simulink model "kaskadydolinearyzacjimud6"  (R2019b)
settings: Solver=VariableStepAuto  StartTime=0.0  StopTime=150  RelTol=1e-3
values from neighbouring files (symbols this model uses):
  A1 = 1    [linearyzacjamud6.m]
  a1 = Aw1*sqrt(2*g)    [linearyzacjamud6.m]
  A2 = 1    [linearyzacjamud6.m]
  a2 = Aw2*sqrt(2*g)    [linearyzacjamud6.m]
  fwe = 0.7*fwemax    [linearyzacjamud6.m]
  fwe0 = 0.1*fwemax    [linearyzacjamud6.m]
  h1pocz = fwe0/a1    [linearyzacjamud6.m]
  h2pocz = fwe0/a2    [linearyzacjamud6.m]
settings Model: Creator=tomek  LastModifiedBy=tomek

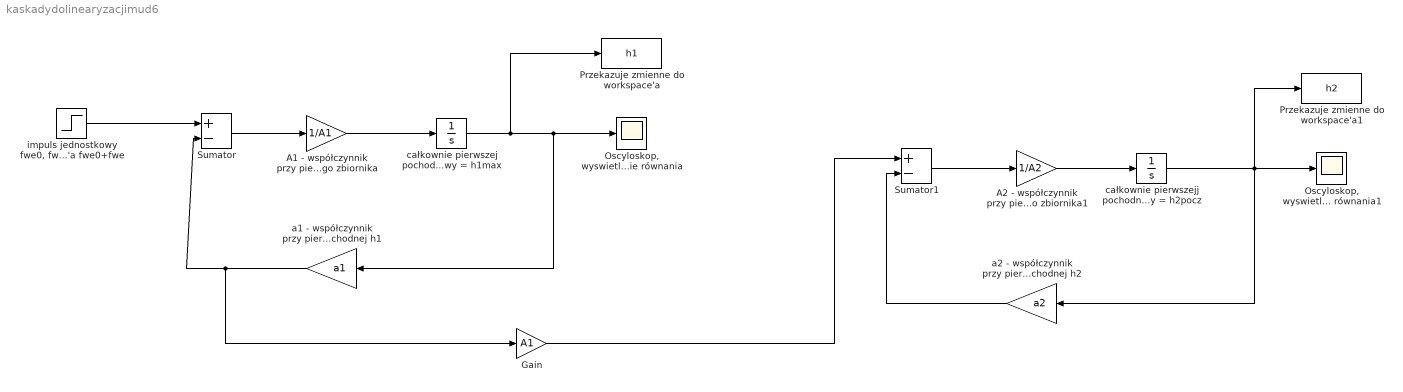
== system kaskadydolinearyzacjimud6 ==
  " całkownie pierwszej pochodnej h1, zawiera warunki początkowe warunek początkowy = h1max" : Integrator  InitialCondition=h1pocz
  " całkownie pierwszejj pochodnej h2 zawiera warunki początkowe warunek poczatkowy = h2pocz" : Integrator  InitialCondition=h2pocz
  A1 - współczynnik przy pierwszej pchodnej h1 Powierzchnia dna pierwszego zbiornika : Gain  Gain=1/A1
  A2 - współczynnik przy pierwszej pchodnej h2 Powierzchnia dna pierwszego zbiornika1 : Gain  Gain=1/A2
  Gain : Gain  Gain=A1
  "Oscyloskop, wyswietla roziwązanie równania" : Scope
  "Oscyloskop, wyswietla roziwązanie równania1" : Scope
  Przekazuje zmienne do workspace'a : ToWorkspace  VariableName=h1  SampleTime=-1
  Przekazuje zmienne do workspace'a1 : ToWorkspace  VariableName=h2  SampleTime=-1
  Sumator : Sum  Inputs=+-
  Sumator1 : Sum  Inputs=+-
  a1 - współczynnik przy pierwszej pochodnej h1 : Gain  Gain=a1
  a2 - współczynnik przy pierwszej pochodnej h2 : Gain  Gain=a2
  "impuls jednostkowy fwe0, fwe - określone w workspace'a fwe0+fwe" : Step  Time=25  Before=fwe0  After=fwe  SampleTime=0
  wires:
  a1 - współczynnik przy pierwszej pochodnej h1/1 -> Gain/1, Sumator/2
  A1 - współczynnik przy pierwszej pchodnej h1 Powierzchnia dna pierwszego zbiornika/1 -> " całkownie pierwszej pochodnej h1, zawiera warunki początkowe warunek początkowy = h1max"/1
  a2 - współczynnik przy pierwszej pochodnej h2/1 -> Sumator1/2
  Sumator/1 -> A1 - współczynnik przy pierwszej pchodnej h1 Powierzchnia dna pierwszego zbiornika/1
  "impuls jednostkowy fwe0, fwe - określone w workspace'a fwe0+fwe"/1 -> Sumator/1
  Sumator1/1 -> A2 - współczynnik przy pierwszej pchodnej h2 Powierzchnia dna pierwszego zbiornika1/1
  Gain/1 -> Sumator1/1
  A2 - współczynnik przy pierwszej pchodnej h2 Powierzchnia dna pierwszego zbiornika1/1 -> " całkownie pierwszejj pochodnej h2 zawiera warunki początkowe warunek poczatkowy = h2pocz"/1
  " całkownie pierwszej pochodnej h1, zawiera warunki początkowe warunek początkowy = h1max"/1 -> Przekazuje zmienne do workspace'a/1, a1 - współczynnik przy pierwszej pochodnej h1/1, "Oscyloskop, wyswietla roziwązanie równania"/1
  " całkownie pierwszejj pochodnej h2 zawiera warunki początkowe warunek poczatkowy = h2pocz"/1 -> a2 - współczynnik przy pierwszej pochodnej h2/1, Przekazuje zmienne do workspace'a1/1, "Oscyloskop, wyswietla roziwązanie równania1"/1
